simulink model "motor_testbench"  (R2021a)
settings: Solver=ode23t  StartTime=0.0  StopTime=0.1  RelTol=1e-3  AbsTol=1e-3  EnableMultiTasking=on
values from neighbouring files (symbols this model uses):
  f = n_rpm/60.0*p    (= 250)    [uz_6ph_pu_vsd_voltages_init.m]    (also in uz_mpc_6ph_init.m; uz_mpc_6ph_state_machine_init.m = 83.3333333333)
  IB = sqrt(2)*IR    [uz_6ph_pu_vsd_voltages_init.m]    (also in uz_mpc_6ph_init.m; uz_mpc_6ph_state_machine_init.m)
  id_ref = 0.0    (= 0)    [uz_6ph_pu_vsd_voltages_init.m]    (also in uz_mpc_6ph_init.m; uz_mpc_6ph_state_machine_init.m)
  iq_ref = -10.0    (= -10)    [uz_6ph_pu_vsd_voltages_init.m]    (also in uz_mpc_6ph_init.m; uz_mpc_6ph_state_machine_init.m = 5)
  ix_ref = 0.0    (= 0)    [uz_6ph_pu_vsd_voltages_init.m]    (also in uz_mpc_6ph_init.m; uz_mpc_6ph_state_machine_init.m)
  iy_ref = 0.0    (= 0)    [uz_6ph_pu_vsd_voltages_init.m]    (also in uz_mpc_6ph_init.m; uz_mpc_6ph_state_machine_init.m)
  lambda_d = 1.0    (= 1)    [uz_mpc_6ph_state_machine_init.m]
  lambda_q = 1.0    (= 1)    [uz_mpc_6ph_state_machine_init.m]
  lambda_u = 0.0    (= 0)    [uz_mpc_6ph_state_machine_init.m]
  lambda_x = 1.0    (= 1)    [uz_mpc_6ph_state_machine_init.m]
  lambda_y = 1.0    (= 1)    [uz_mpc_6ph_state_machine_init.m]
  Ld_over_LB = Ld/LB    [uz_6ph_pu_vsd_voltages_init.m]    (also in uz_mpc_6ph_init.m; uz_mpc_6ph_state_machine_init.m)
  Lq_over_LB = Lq/LB    [uz_6ph_pu_vsd_voltages_init.m]    (also in uz_mpc_6ph_init.m; uz_mpc_6ph_state_machine_init.m)
  omega_m = n_rpm*pi/30    (= 314.159265359)    [uz_6ph_pu_vsd_voltages_init.m]    (also in uz_mpc_6ph_init.m; uz_mpc_6ph_state_machine_init.m = 104.71975512)
  omegaB = nR*2*pi()/60*p    [uz_6ph_pu_vsd_voltages_init.m]    (also in uz_mpc_6ph_init.m; uz_mpc_6ph_state_machine_init.m)
  p = 5    [uz_6ph_pu_vsd_voltages_init.m]    (also in uz_mpc_6ph_init.m; uz_mpc_6ph_state_machine_init.m)
  psi_pm_over_psiB = psi_pm/psiB    [uz_6ph_pu_vsd_voltages_init.m]    (also in uz_mpc_6ph_init.m; uz_mpc_6ph_state_machine_init.m)
  Rs_over_ZB = Rs/ZB    [uz_6ph_pu_vsd_voltages_init.m]    (also in uz_mpc_6ph_init.m; uz_mpc_6ph_state_machine_init.m)
  t_ADC = 1/f_ADC    (= 1e-05)    [uz_6ph_pu_vsd_voltages_init.m]    (also in uz_mpc_6ph_init.m; uz_mpc_6ph_state_machine_init.m; uz_typeconv_init.m)
  t_clock = 1/f_clock    (= 1e-08)    [uz_6ph_pu_vsd_voltages_init.m]    (also in uz_mpc_6ph_init.m; uz_mpc_6ph_state_machine_init.m; uz_typeconv_init.m)
  Ts_times_ZB_over_Ld = Ts*ZB/Ld    [uz_6ph_pu_vsd_voltages_init.m]    (also in uz_mpc_6ph_init.m; uz_mpc_6ph_state_machine_init.m)
  Ts_times_ZB_over_Lq = Ts*ZB/Lq    [uz_6ph_pu_vsd_voltages_init.m]    (also in uz_mpc_6ph_init.m; uz_mpc_6ph_state_machine_init.m)
  Ts_times_ZB_over_Lx = Ts*ZB/Lx    [uz_6ph_pu_vsd_voltages_init.m]    (also in uz_mpc_6ph_init.m; uz_mpc_6ph_state_machine_init.m)
  Ts_times_ZB_over_Ly = Ts*ZB/Ly    [uz_6ph_pu_vsd_voltages_init.m]    (also in uz_mpc_6ph_init.m; uz_mpc_6ph_state_machine_init.m)
  v_dc = 565.0    (= 565)    [uz_6ph_pu_vsd_voltages_init.m]    (also in uz_mpc_6ph_init.m; uz_mpc_6ph_state_machine_init.m)
  VB = sqrt(2/3)*VR    [uz_6ph_pu_vsd_voltages_init.m]    (also in uz_mpc_6ph_init.m; uz_mpc_6ph_state_machine_init.m)
undefined symbols (not defined in the file or in its folder): Newton, Raphson
libraries: nesl_utility x33, fl_lib x26, ee_lib x12, simulink x10, hdlsllib x2, spsAlphaBetaZerotodq0Lib x1
(part 1 of 3)
settings Model: Creator=Michael Hoerner  LastModifiedBy=micha
settings SolverCC: AutoScaleAbsTol=off  AlgebraicLoopSolver=TrustRegion  DecoupledContinuousIntegration=on  MinimalZcImpactIntegration=on
settings DataIOCC: LimitDataPoints=on  MaxDataPoints=10000  ReturnWorkspaceOutputs=off
settings OptimizationCC: DefaultParameterBehavior=Inlined  PassReuseOutputArgsAs=Individual arguments  OptimizeBlockOrder=speed  DifferentSizesBufferReuse=on  EfficientTunableParamExpr=on
settings DebuggingCC: ParameterTunabilityLossMsg=error  AllowSymbolicDim=off  SFUnexpectedBacktrackingDiag=warning  SFNoUnconditionalDefaultTransitionDiag=warning  SFExecutionAtInitializationDiag=none  SFMachineParentedDataDiag=warning  ArithmeticOperatorsInVariantConditions=warning
settings HardwareCC: ProdBitPerPointer=32  ProdBitPerSizeT=32  ProdBitPerPtrDiffT=32  ProdLargestAtomicInteger=Long  ProdLargestAtomicFloat=Double  ProdWordSize=32  ProdHWDeviceType=ARM Compatible->ARM Cortex-R
settings SFSimCC: SimUseLocalCustomCode=off  MATLABDynamicMemAlloc=off  CustomCodeUndefinedFunction=UseInterfaceOnly
settings RTWCC: SystemTargetFile=ert.tlc  GenCodeOnly=on  TemplateMakefile=ert_default_tmf  GenerateReport=on  RTWUseLocalCustomCode=off  BuildConfiguration=Faster Runs  IncludeHyperlinkInReport=on  GenerateTraceInfo=on  GenerateTraceReport=on  GenerateTraceReportSl=on  GenerateTraceReportSf=on  GenerateTraceReportEml=on  GenerateCodeMetricsReport=on  CheckMdlBeforeBuild=Warning
settings CodeAppCC: ForceParamTrailComments=on  IgnoreCustomStorageClasses=off  OperatorAnnotations=on  SimulinkDataObjDesc=on  SFDataObjDesc=on  MATLABFcnDesc=on  InsertBlockDesc=on  StateflowObjectComments=on  MATLABSourceComments=on  EnableCustomComments=on  ReqsInCode=on
settings ERTTargetCC: CodeReplacementLibrary=GNU C99 extensions  GenerateSampleERTMain=on  SuppressErrorStatus=on  IncludeFileDelimiter=UseQuote  CodeInterfacePackaging=Reusable function  SupportNonFinite=off  MultiInstanceErrorCode=Warning  RootIOFormat=Part of model data structure  ERTCustomFileTemplate=example_file_process.tlc  GlobalDataDefinition=InSourceFile  GlobalDataReference=InSourceFile  ERTFilePackagingFormat=CompactWithDataFile
settings ConfigComp: CovMetricSettings=dw  CovSaveCumulativeToWorkspaceVar=on  CovSaveSingleToWorkspaceVar=on  CovExternalEMLEnable=off  CovSFcnEnable=off
settings SimscapeCC: SimscapeLogDataHistory=10000

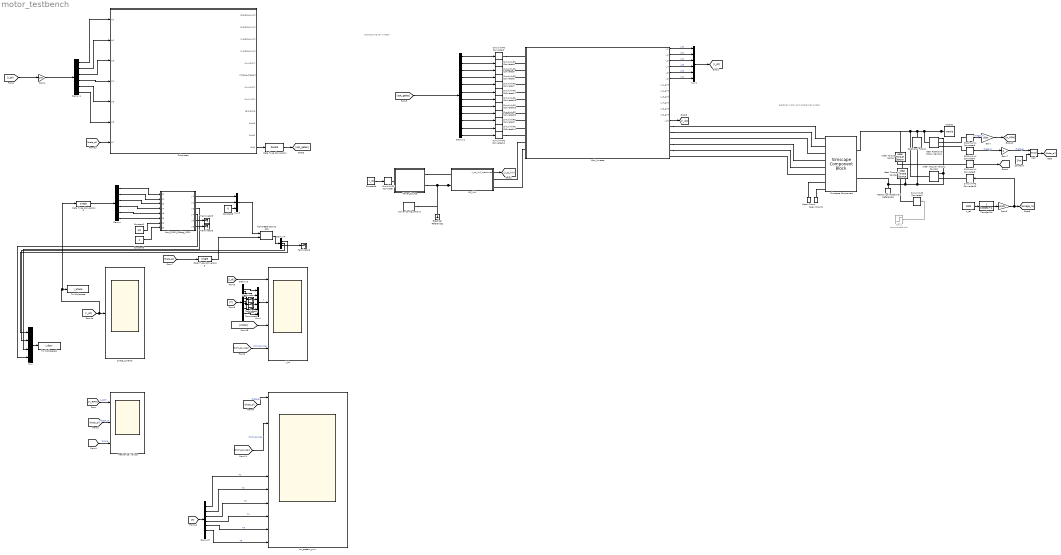
== system motor_testbench ==
  note: electrical motor and mechanical system
  note: 6-phase 2-level inverter
  6ph_Inverter : Subsystem
  6ph_PMSM_30deg_VSD1 : MATLAB Function  TreatAsAtomicUnit=on
  Alpha-Beta-Zero to dq0 : spsAlphaBetaZerotodq0Lib/Alpha-Beta-Zero to dq0  Alignment=Aligned with phase A axis
      settings: SourceProductBaseCode=PS
  Constant : Constant  Value=2*pi
  Constant1 : Constant  Value=1/3
  Constant6 : Constant  Value=v_dc
  Constant8 : Constant  Value=0  OutDataTypeStr=single
  Constant9 : Constant
  DC_link : Subsystem
  Data Type Conversion : DataTypeConversion  OutDataTypeStr=double  LockScale=on
  Data Type Conversion5 : DataTypeConversion  OutDataTypeStr=single
  Data Type Conversion6 : DataTypeConversion  OutDataTypeStr=single
  Demux : Demux  Outputs=6
  Demux1 : Demux  Outputs=6
  Demux2 : Demux  Outputs=12
  Demux3 : Demux  Outputs=12
  Demux4 : Demux  Outputs=3
  Demux5 : Demux  Outputs=12
  Electrical Reference1 : fl_lib/Electrical/Electrical Elements/Electrical Reference
  Gain : Gain  Gain=30/pi
  Gain1 : Gain  Gain=1/IB
  Gain7 : Gain  Gain=p
  Gain8 : Gain  Gain=pi/30
  Ideal Angular Velocity Source1 : fl_lib/Mechanical/Mechanical Sources/Ideal Angular Velocity Source
  Ideal Rotational Motion Sensor1 : fl_lib/Mechanical/Mechanical Sensors/Ideal Rotational Motion Sensor  wrap_angle=simscape.enum.onoff.off  offset=0 deg
  Ideal Torque Sensor : fl_lib/Mechanical/Mechanical Sensors/Ideal Torque Sensor
  Ideal Torque Source : fl_lib/Mechanical/Mechanical Sources/Ideal Torque Source
  Inertia1 : fl_lib/Mechanical/Rotational Elements/Inertia  inertia=J kg*m^2  num_ports=foundation.enum.numPorts2.one  w_specify=off  w_priority=High  w=0 rad/s  w_nominal_specify=off  w_nominal_unit=rad/s  w_nominal_value=1  t_specify=off  t_priority=None  t=0 N*m  t_nominal_specify=off  t_nominal_unit=N*m  t_nominal_value=1
  Mechanical Rotational Reference1 : fl_lib/Mechanical/Rotational Elements/Mechanical Rotational Reference
  Mod : Math  Operator=mod  SaturateOnIntegerOverflow=on
  Mux : Mux
  Mux1 : Mux  Inputs=6
  Mux4 : Mux  Inputs=6
  Mux5 : Mux  Inputs=3
  Open Circuit : fl_lib/Electrical/Electrical Elements/Open Circuit  v_specify=off  v_priority=None  v=0 V  v_nominal_specify=off  v_nominal_unit=V  v_nominal_value=1
      settings: SourceProductBaseCode=SS
  Open Circuit1 : fl_lib/Electrical/Electrical Elements/Open Circuit  v_specify=off  v_priority=None  v=0 V  v_nominal_specify=off  v_nominal_unit=V  v_nominal_value=1
      settings: SourceProductBaseCode=SS
  PS-Simulink Converter6 : nesl_utility/PS-Simulink Converter  PhysicalDomain=network_engine_domain  SubClassName=ps_output  LeftPortType=input  RightPortType=output  PseudoPeriodic=off  Frequencies=[]  Unit=1  AffineConversion=off
      settings: SourceProductBaseCode=PW,SS
  PS-Simulink Converter7 : nesl_utility/PS-Simulink Converter  PhysicalDomain=network_engine_domain  SubClassName=ps_output  LeftPortType=input  RightPortType=output  PseudoPeriodic=off  Frequencies=[]  Unit=1  AffineConversion=off
      settings: SourceProductBaseCode=PW,SS
  PS-Simulink Converter8 : nesl_utility/PS-Simulink Converter  PhysicalDomain=network_engine_domain  SubClassName=ps_output  LeftPortType=input  RightPortType=output  PseudoPeriodic=off  Frequencies=[]  Unit=1  AffineConversion=off
      settings: SourceProductBaseCode=PW,SS
  Power_Source : Subsystem
  Rotational Friction : fl_lib/Mechanical/Rotational Elements/Rotational Friction  brkwy_trq=0.0622476 N*m  brkwy_vel=0.1 rad/s  Col_trq=0.03460117 N*m  visc_coef=0.00026373 N*m/(rad/s)  w_specify=off  w_priority=None  w=0 rad/s  w_nominal_specify=off  w_nominal_unit=rad/s  w_nominal_value=1  t_specify=off  t_priority=None  t=0 N*m  t_nominal_specify=off  t_nominal_unit=N*m  t_nominal_value=1
  Simscape Component : SimscapeComponentBlock  SourceFile=SixPhase_PMSM  ComponentPath=SixPhase_PMSM  ComponentVariants=SixPhase_PMSM  ComponentVariantNames=SixPhase_PMSM  ClassName=SixPhase_PMSM  SchemaVersion=1  Rs=Rs Ohm  Ld=Ld H  Lq=Lq H  Lx=Lx H  Ly=Ly H  psiPM=psi_pm Wb  np=p  theta_m_specify=off  theta_m_priority=None  theta_m=0 rad  theta_m_nominal_specify=off  theta_m_nominal_unit=rad  theta_m_nominal_value=1
      settings: CopyFcn=simscape.engine.sli.internal.componentblockcallback(gcbh,'COPY')  PreCopyFcn=simscape.engine.sli.internal.componentblockcallback(gcbh,'PRECOPY')  PreDeleteFcn=simscape.engine.sli.internal.componentblockcallback(gcbh,'PREDELETE')  InternalSimscapePortConfiguration="{\"Bottom\":[],\"Left\":[{\"id\":\"a1\",\"label\":\"a1\",\"type\":\"foundation.electrical.electrical\"},{\"id\":\"b1\",\"label\":\"b1\",\"type\":\"foundation.electrical.electrical\"},{\"id\":\"c1\",\"label\":\"c1\",\"type\":\"foundation.electrical.electrical\"},{\"id\":\"a2\",\"label\":\"a2\",\"type\":\"foundation.electrical.electrical\"},{\"id\":\"b2\",\"label\":\"b2\",\"type\":\"foundation.electrical.electrical\"},{\"id\":\"c2\",\"label\":\"c2\",\"type\":\"foundation.electrical.electrical\"},{\"id\":\"n1\",\"label\":\"n1\",\"type\":\"foundation.electrical.electrical\"},{\"id\":\"n2\",\"label\":\"n2\",\"type\":\"foundation.electrical.electrical\"}],\"Right\":[{\"id\":\"R\",\"label\":\"R\",\"type\":\"foundation.mechanical.rotational.rotational\"},{\"id\":\"C\",\"label\":\"C\",\"type\":\"foundation.mechanical.rotational.rotational\"}],\"Top\":[]}"
      mask Type: SixPhase_PMSM
  Simulink-PS Converter{,2..7,11..12,17..20} (13 alike) : nesl_utility/Simulink-PS Converter  PhysicalDomain=network_engine_domain  SubClassName=ps_input  LeftPortType=input  RightPortType=output  PseudoPeriodic=off  Frequencies=[]  NoiseDistribution=none  NoiseParameters=[]  Unit=1  AffineConversion=off  FilteringAndDerivatives=provide  SimscapeFilterOrder=1  InputFilterTimeConstant=0.001  UdotUserProvided=0
      Simulink-PS Converter settings: SourceProductBaseCode=PW,SS
  Simulink-PS Converter1 : nesl_utility/Simulink-PS Converter  PhysicalDomain=network_engine_domain  SubClassName=ps_input  LeftPortType=input  RightPortType=output  PseudoPeriodic=off  Frequencies=[]  NoiseDistribution=none  NoiseParameters=[]  Unit=1  AffineConversion=off  FilteringAndDerivatives=filter  SimscapeFilterOrder=1  InputFilterTimeConstant=0.001  UdotUserProvided=0
      settings: SourceProductBaseCode=PW,SS
  Simulink-PS Converter10 : nesl_utility/Simulink-PS Converter  PhysicalDomain=network_engine_domain  SubClassName=ps_input  LeftPortType=input  RightPortType=output  PseudoPeriodic=off  Frequencies=[]  NoiseDistribution=none  NoiseParameters=[]  Unit=1  AffineConversion=off  FilteringAndDerivatives=filter  SimscapeFilterOrder=1  InputFilterTimeConstant=0.001  UdotUserProvided=0
      settings: SourceProductBaseCode=PW,SS
  Solver Configuration1 : nesl_utility/Solver Configuration  PhysicalDomain=network_engine_domain  SubClassName=solver  LeftPortType=input  RightPortType=generic  Tones=[]  Harmonics=[]  SimulateNoise=off  Profile=off  UseLocalSampling=off  EnableSwitchedLinearOptims=on  FrequencyDomain=off  UseCCode=off  RelTol=0.001  AbsTol=1e-06  MinStep=1e-09  ToWorkspace=off  RevertToSquareIcSolve=off  NumHomotopyIterations=100  PhasorMode=off  PhasorModeNumHarmonics=1  DoDC=off  ResidualTolerance=1e-09  UseLocalSolver=off  LocalSolverChoice=NE_BACKWARD_EULER_ADVANCER  LocalSolverSampleTime=1e-6  DoFixedCost=off  MaxNonlinIter=3  MaxModeIter=2  ComputeImpulses=off  ImpulseIterations=2  LinearAlgebra=Sparse  EquationFormulation=NE_TIME_EF  DelaysMemoryBudget=1024  AutomaticFiltering=on  FilteringTimeConstant=0.001  PartitionStorageMethod=AS_NEEDED  PartitionMemoryBudget=1024  PartitionMethod=FAST
      settings: SourceProductBaseCode=PW,SS
  Step1 : Step  Commented=on  Time=0.08  After=-0.5  SampleTime=0
  Subsystem : Subsystem
  Terminator{,1..3,5..6} (6 alike) : Terminator
  To Workspace : ToWorkspace  VariableName=i_phase  SaveFormat=Timeseries  SampleTime=1e-6
  To Workspace1 : ToWorkspace  VariableName=i_dqxy  SaveFormat=Timeseries  SampleTime=50e-6
  Transfer Fcn : TransferFcn  Denominator=[0.0005 1]
  i_dc : Scope  NumInputPorts=4
  mechanical values : Scope  NumInputPorts=3
  n_ref : Constant  Value=1000
  phase_currents : Scope
  sw_pattern_svm : Scope  NumInputPorts=12
  wires:
  DC_link/1(u_dc_link_measured) -> [u_dc_link]
  Constant6/1 -> Simulink-PS Converter/1
  PS-Simulink Converter7/1 -> Gain7/1  "theta_m"
  Gain7/1 -> Mod/1  "theta_el"
  Gain8/1 -> Simulink-PS Converter10/1, [omega_m]
  PS-Simulink Converter6/1 -> Gain/1  "omega_m"
  PS-Simulink Converter8/1 -> [torque]
  [T] -> Demux3/1
  Demux3/1 -> Mux4/1
  Demux3/3 -> Mux4/2
  Demux3/5 -> Mux4/3
  Demux3/2 -> Terminator/1
  Demux3/4 -> Terminator1/1
  [PWM_counter] -> i_dc/4  "PWM_counter"
  [i_dc] -> i_dc/1
  Demux3/6 -> Terminator3/1
  [i_ph] -> Data Type Conversion6/1, To Workspace/1, phase_currents/1
  Mux4/1 -> i_dc/2  "T"
  n_ref/1 -> Transfer Fcn/1
  Transfer Fcn/1 -> Gain8/1
  [CMPA] -> i_dc/3
  Gain/1 -> [n_RPM]
  Step1/1 -> Simulink-PS Converter1/1
  [torque] -> mechanical values/3  "torque"
  [n_RPM] -> mechanical values/1  "n_RPM"
  [theta_el] -> mechanical values/2  "theta_el"
  6ph_Inverter/1(i_1) -> Mux1/1  "i_a1"
  6ph_Inverter/6(i_6) -> Mux1/6  "i_c2"
  6ph_Inverter/4(i_4) -> Mux1/4  "i_a2"
  Demux2/6 -> Simulink-PS Converter17/1
  Demux2/5 -> Simulink-PS Converter7/1
  6ph_Inverter/13(i_dc) -> [i_dc]
  Demux2/7 -> Simulink-PS Converter18/1
  6ph_Inverter/3(i_3) -> Mux1/3  "i_c1"
  6ph_Inverter/5(i_5) -> Mux1/5  "i_b2"
  Demux2/3 -> Simulink-PS Converter5/1
  6ph_Inverter/2(i_2) -> Mux1/2  "i_b1"
  Demux2/2 -> Simulink-PS Converter4/1
  Demux2/11 -> Simulink-PS Converter11/1
  Demux2/12 -> Simulink-PS Converter12/1
  Demux2/8 -> Simulink-PS Converter19/1
  Demux2/9 -> Simulink-PS Converter20/1
  Demux2/4 -> Simulink-PS Converter6/1
  Demux2/10 -> Simulink-PS Converter3/1
  Demux2/1 -> Simulink-PS Converter2/1
  Mux1/1 -> [i_ph]
  Constant/1 -> Mod/2
  Mod/1 -> [theta_el]
  Mux/1 -> To Workspace1/1
  6ph_PMSM_30deg_VSD1/3(y3) -> Mux/3
  Demux/2 -> 6ph_PMSM_30deg_VSD1/2(u2)
  Constant8/1 -> Mux5/3
  Constant9/1 -> 6ph_PMSM_30deg_VSD1/8(c6)
  Demux/5 -> 6ph_PMSM_30deg_VSD1/5(u5)
  Demux/4 -> 6ph_PMSM_30deg_VSD1/4(u4)
  Demux/6 -> 6ph_PMSM_30deg_VSD1/6(u6)
  6ph_PMSM_30deg_VSD1/2(y2) -> Mux5/2
  6ph_PMSM_30deg_VSD1/6(y6) -> Terminator6/1
  Demux/3 -> 6ph_PMSM_30deg_VSD1/3(u3)
  Constant1/1 -> 6ph_PMSM_30deg_VSD1/7(k6)
  Demux/1 -> 6ph_PMSM_30deg_VSD1/1(u1)
  6ph_PMSM_30deg_VSD1/4(y4) -> Mux/4
  Mux5/1 -> Alpha-Beta-Zero to dq0/1
  6ph_PMSM_30deg_VSD1/5(y5) -> Terminator5/1
  6ph_PMSM_30deg_VSD1/1(y1) -> Mux5/1
  [theta_el] -> Data Type Conversion5/1
  Alpha-Beta-Zero to dq0/1 -> Demux4/1
  Demux4/1 -> Mux/1
  Demux4/2 -> Mux/2
  Demux4/3 -> Terminator2/1
  Data Type Conversion5/1 -> Alpha-Beta-Zero to dq0/2
  Data Type Conversion6/1 -> Demux/1
  Demux3/11 -> Mux4/6
  Demux3/9 -> Mux4/5
  Demux3/7 -> Mux4/4
  [theta_el] -> sw_pattern_svm/1  "theta_el"
  [PWM_counter] -> sw_pattern_svm/3  "PWM_counter"
  Demux5/7 -> sw_pattern_svm/10  "T4"
  Demux5/3 -> sw_pattern_svm/8  "T2"
  Demux5/9 -> sw_pattern_svm/11  "T5"
  [T] -> Demux5/1
  Demux5/1 -> sw_pattern_svm/7  "T1"
  Demux5/5 -> sw_pattern_svm/9  "T3"
  Demux5/11 -> sw_pattern_svm/12  "T6"
  [opt_gates] -> Demux2/1
  Subsystem/12(Out1) -> Data Type Conversion/1
  Data Type Conversion/1 -> [opt_gates]
  Demux1/1 -> Subsystem/1(In1)
  [i_ph] -> Gain1/1
  Gain1/1 -> Demux1/1
  Demux1/2 -> Subsystem/2(In2)
  Demux1/3 -> Subsystem/3(In3)
  Demux1/4 -> Subsystem/4(In4)
  Demux1/5 -> Subsystem/5(In5)
  Demux1/6 -> Subsystem/6(In6)
  [theta_el] -> Subsystem/7(In7)
  connections:
  DC_link/LConn2 -- Power_Source/RConn2 -- Solver Configuration1/RConn1 -- Electrical Reference1/LConn1
  Inertia1/LConn1 -- Ideal Torque Sensor/LConn1 -- Simscape Component/RConn1 -- Ideal Angular Velocity Source1/LConn1 -- Rotational Friction/LConn1 -- Ideal Rotational Motion Sensor1/LConn1
  Ideal Rotational Motion Sensor1/RConn1 -- Ideal Angular Velocity Source1/RConn2 -- Rotational Friction/RConn1 -- Simscape Component/RConn2 -- Mechanical Rotational Reference1/LConn1 -- Ideal Torque Source/RConn2
  Power_Source/RConn1 -- DC_link/LConn1
  PS-Simulink Converter6/LConn1 -- Ideal Rotational Motion Sensor1/RConn2
  Simulink-PS Converter/RConn1 -- Power_Source/LConn1
  6ph_Inverter/LConn13 -- DC_link/RConn1
  6ph_Inverter/LConn14 -- DC_link/RConn2
  PS-Simulink Converter7/LConn1 -- Ideal Rotational Motion Sensor1/RConn3
  Simulink-PS Converter10/RConn1 -- Ideal Angular Velocity Source1/RConn1
  PS-Simulink Converter8/LConn1 -- Ideal Torque Sensor/RConn2
  Simulink-PS Converter1/RConn1 -- Ideal Torque Source/RConn1
  Ideal Torque Source/LConn1 -- Ideal Torque Sensor/RConn1
  Simscape Component/LConn8 -- Open Circuit1/LConn1
  6ph_Inverter/RConn2 -- Simscape Component/LConn2
  Simscape Component/LConn7 -- Open Circuit/LConn1
  6ph_Inverter/RConn1 -- Simscape Component/LConn1
  6ph_Inverter/RConn4 -- Simscape Component/LConn4
  6ph_Inverter/RConn5 -- Simscape Component/LConn5
  Simulink-PS Converter7/RConn1 -- 6ph_Inverter/LConn5
  Simulink-PS Converter12/RConn1 -- 6ph_Inverter/LConn12
  Simulink-PS Converter20/RConn1 -- 6ph_Inverter/LConn9
  Simulink-PS Converter17/RConn1 -- 6ph_Inverter/LConn6
  Simulink-PS Converter11/RConn1 -- 6ph_Inverter/LConn11
  Simulink-PS Converter19/RConn1 -- 6ph_Inverter/LConn8
  Simulink-PS Converter6/RConn1 -- 6ph_Inverter/LConn4
  Simulink-PS Converter3/RConn1 -- 6ph_Inverter/LConn10
  Simulink-PS Converter4/RConn1 -- 6ph_Inverter/LConn2
  Simscape Component/LConn3 -- 6ph_Inverter/RConn3
  Simscape Component/LConn6 -- 6ph_Inverter/RConn6
  Simulink-PS Converter5/RConn1 -- 6ph_Inverter/LConn3
  Simulink-PS Converter2/RConn1 -- 6ph_Inverter/LConn1
  Simulink-PS Converter18/RConn1 -- 6ph_Inverter/LConn7

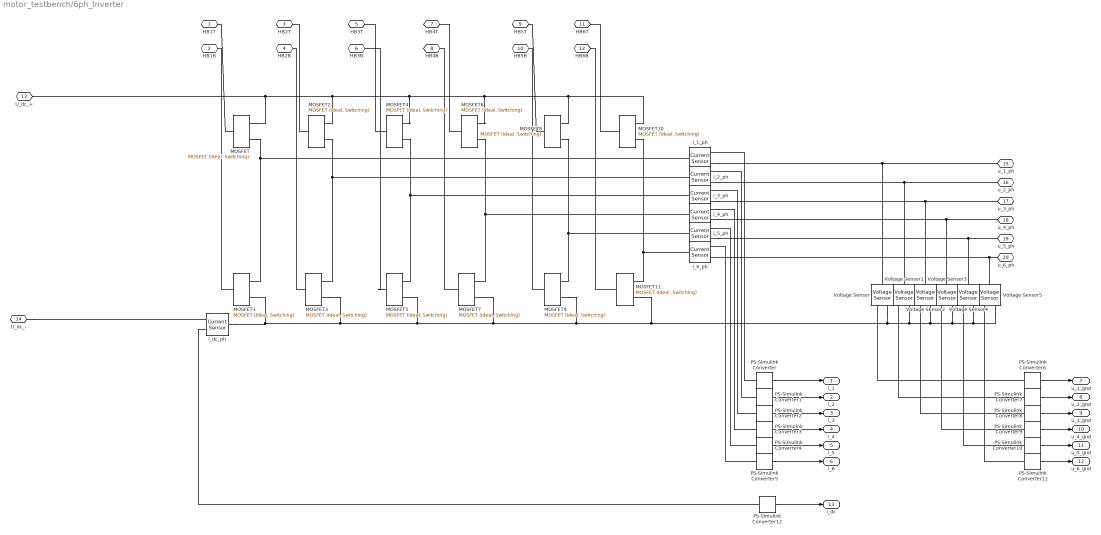
== system motor_testbench/6ph_Inverter ==
  MOSFET{,1..11} (12 alike) : ee_lib/Semiconductors & Converters/MOSFET (Ideal, Switching)  Rds=RDSon Ohm  Goff=1e-6 1/Ohm  Vth=0.7 V  diode_param=1  diode_Vf=0.8 V  diode_Ron=0.001 Ohm  diode_Goff=1e-5 1/Ohm  diode_C=5e-8 F  diode_iRM=-235 A  diode_iF=300 A  diode_idot=-50 A/us  diode_trr_param=1  diode_trr_factor=3  diode_trr=15 us  diode_Qrr=1.5e+3 s*uA  thermal_loss_option=ee.enum.converters.thermalLossOption.constantvalues  Von_data=[0, 1.1, 1.3, 1.45, 1.75, 2.25, 2.7; 0, 1, 1.15, 1.35, 1.7, 2.35, 3] V  Eon_data=[0, .29, 1.43, 2.86, 5.71, 13.14, 22.86; 0, .57, 2.63, 5.14, 10.29, 20.57, 30.29] * 1e-3 J  Eoff_data=[0, .21, 1.07, 2.14, 4.29, 9.86, 17.14; 0, .43, 1.97, 3.86, 7.71, 15.43, 22.71] * 1e-3 J  Tj=[298.15, 398.15] K  Iout_data=[0, 10, 50, 100, 200, 400, 600] A  Eon_scalar=22.86e-3 J  Eoff_scalar=17.14e-3 J  Voff=300 V  Iout_scalar=600 A  diodeModelType=ee.enum.converters.diodeModelType.pwl  diode_IfMat=[.07, .12, .19, 1.75, 4.24, 7.32, 11.2; .16, .3, .72, 2.14, 4.02, 6.35, 9.12] A  diode_TjVec=[25, 125] degC  diode_VfVec=[.5, .7, .9, 1.3, 1.7, 2.1, 2.5] V  thermal_network_parameterization=ee.enum.thermalNetworkTopology.external  Rth=[.03, .2] K/W  Rth_Foster=[.03, .2] K/W  thermal_mass_parameterization=ee.enum.thermalNetwork.timeconstant  thermal_mass=[3, 25] J/K  thermal_mass_Foster=[33, 50] J/K  thermal_time_constant=[.1, 5] s  thermal_time_constant_Foster=[1, 10] s  thermal_mass_initial_temperatures=[25, 25] degC  junction_thermal_mass=0.1 J/K  vT_specify=off  vT_priority=None  vT=0 V  vT_nominal_specify=off  vT_nominal_unit=V  vT_nominal_value=1  Qj_specify=off  Qj_priority=None  Qj=0 W  Qj_nominal_specify=off  Qj_nominal_unit=W  Qj_nominal_value=1  junction_temperature_specify=off  junction_temperature_priority=None  junction_temperature=25 degC  junction_temperature_nominal_specify=off  junction_temperature_nominal_unit=degC  junction_temperature_nominal_value=1
  PS-Simulink Converter{,1..5,12} (7 alike) : nesl_utility/PS-Simulink Converter  PhysicalDomain=network_engine_domain  SubClassName=ps_output  LeftPortType=input  RightPortType=output  PseudoPeriodic=off  Frequencies=[]  Unit=A  AffineConversion=off
  PS-Simulink Converter{6..11} (6 alike) : nesl_utility/PS-Simulink Converter  PhysicalDomain=network_engine_domain  SubClassName=ps_output  LeftPortType=input  RightPortType=output  PseudoPeriodic=off  Frequencies=[]  Unit=V  AffineConversion=off
  Voltage Sensor{,1..5} (6 alike) : fl_lib/Electrical/Electrical Sensors/Voltage Sensor
  i_1_ph : fl_lib/Electrical/Electrical Sensors/Current Sensor
  i_2_ph : fl_lib/Electrical/Electrical Sensors/Current Sensor
  i_3_ph : fl_lib/Electrical/Electrical Sensors/Current Sensor
  i_4_ph : fl_lib/Electrical/Electrical Sensors/Current Sensor
  i_5_ph : fl_lib/Electrical/Electrical Sensors/Current Sensor
  i_6_ph : fl_lib/Electrical/Electrical Sensors/Current Sensor
  i_dc_ph : fl_lib/Electrical/Electrical Sensors/Current Sensor
  HB1T : PMIOPort  Side=Left
  HB1B : PMIOPort  Port=2  Side=Left
  HB2T : PMIOPort  Port=3  Side=Left
  HB2B : PMIOPort  Port=4  Side=Left
  HB3T : PMIOPort  Port=5  Side=Left
  HB3B : PMIOPort  Port=6  Side=Left
  HB4T : PMIOPort  Port=7  Side=Left
  HB4B : PMIOPort  Port=8  Side=Left
  HB5T : PMIOPort  Port=9  Side=Left
  HB5B : PMIOPort  Port=10  Side=Left
  HB6T : PMIOPort  Port=11  Side=Left
  HB6B : PMIOPort  Port=12  Side=Left
  U_dc_+ : PMIOPort  Port=13  Side=Left
  U_dc_- : PMIOPort  Port=14  Side=Left
  u_1_ph : PMIOPort  Port=15  Side=Right
  u_2_ph : PMIOPort  Port=16  Side=Right
  u_3_ph : PMIOPort  Port=17  Side=Right
  u_4_ph : PMIOPort  Port=18  Side=Right
  u_5_ph : PMIOPort  Port=19  Side=Right
  u_6_ph : PMIOPort  Port=20  Side=Right
  i_1 : Outport  VectorParamsAs1DForOutWhenUnconnected=off
  i_2 : Outport  Port=2  VectorParamsAs1DForOutWhenUnconnected=off
  i_3 : Outport  Port=3  VectorParamsAs1DForOutWhenUnconnected=off
  i_4 : Outport  Port=4  VectorParamsAs1DForOutWhenUnconnected=off
  i_5 : Outport  Port=5  VectorParamsAs1DForOutWhenUnconnected=off
  i_6 : Outport  Port=6  VectorParamsAs1DForOutWhenUnconnected=off
  u_1_gnd : Outport  Port=7  VectorParamsAs1DForOutWhenUnconnected=off
  u_2_gnd : Outport  Port=8  VectorParamsAs1DForOutWhenUnconnected=off
  u_3_gnd : Outport  Port=9  VectorParamsAs1DForOutWhenUnconnected=off
  u_4_gnd : Outport  Port=10  VectorParamsAs1DForOutWhenUnconnected=off
  u_5_gnd : Outport  Port=11  VectorParamsAs1DForOutWhenUnconnected=off
  u_6_gnd : Outport  Port=12  VectorParamsAs1DForOutWhenUnconnected=off
  i_dc : Outport  Port=13  VectorParamsAs1DForOutWhenUnconnected=off
  wires:
  PS-Simulink Converter/1 -> i_1/1
  PS-Simulink Converter1/1 -> i_2/1
  PS-Simulink Converter2/1 -> i_3/1
  PS-Simulink Converter3/1 -> i_4/1
  PS-Simulink Converter4/1 -> i_5/1
  PS-Simulink Converter5/1 -> i_6/1
  PS-Simulink Converter9/1 -> u_4_gnd/1
  PS-Simulink Converter8/1 -> u_3_gnd/1
  PS-Simulink Converter7/1 -> u_2_gnd/1
  PS-Simulink Converter6/1 -> u_1_gnd/1
  PS-Simulink Converter10/1 -> u_5_gnd/1
  PS-Simulink Converter11/1 -> u_6_gnd/1
  PS-Simulink Converter12/1 -> i_dc/1
  connections:
  MOSFET6/RConn2 -- i_4_ph/LConn1 -- MOSFET7/RConn1
  MOSFET2/RConn2 -- i_2_ph/LConn1 -- MOSFET3/RConn1
  MOSFET4/RConn2 -- i_3_ph/LConn1 -- MOSFET5/RConn1
  MOSFET5/RConn2 -- Voltage Sensor5/RConn2 -- Voltage Sensor4/RConn2 -- Voltage Sensor3/RConn2 -- Voltage Sensor2/RConn2 -- Voltage Sensor1/RConn2 -- Voltage Sensor/RConn2 -- MOSFET11/RConn2 -- MOSFET9/RConn2 -- MOSFET7/RConn2 -- i_dc_ph/LConn1 -- MOSFET1/RConn2 -- MOSFET3/RConn2
  MOSFET/RConn2 -- i_1_ph/LConn1 -- MOSFET1/RConn1
  MOSFET11/LConn1 -- HB6B/RConn1
  MOSFET8/RConn2 -- i_5_ph/LConn1 -- MOSFET9/RConn1
  MOSFET2/LConn1 -- HB2T/RConn1
  MOSFET10/RConn2 -- i_6_ph/LConn1 -- MOSFET11/RConn1
  MOSFET/LConn1 -- HB1T/RConn1
  MOSFET9/LConn1 -- HB5B/RConn1
  MOSFET5/LConn1 -- HB3B/RConn1
  MOSFET1/LConn1 -- HB1B/RConn1
  MOSFET7/LConn1 -- HB4B/RConn1
  MOSFET8/LConn1 -- HB5T/RConn1
  MOSFET4/LConn1 -- HB3T/RConn1
  MOSFET10/LConn1 -- HB6T/RConn1
  MOSFET6/LConn1 -- HB4T/RConn1
  MOSFET3/LConn1 -- HB2B/RConn1
  i_1_ph/RConn2 -- Voltage Sensor/LConn1 -- u_1_ph/RConn1
  i_2_ph/RConn2 -- u_2_ph/RConn1 -- Voltage Sensor1/LConn1
  i_3_ph/RConn2 -- u_3_ph/RConn1 -- Voltage Sensor2/LConn1
  i_4_ph/RConn2 -- Voltage Sensor3/LConn1 -- u_4_ph/RConn1
  i_5_ph/RConn2 -- Voltage Sensor4/LConn1 -- u_5_ph/RConn1
  u_6_ph/RConn1 -- i_6_ph/RConn2 -- Voltage Sensor5/LConn1
  PS-Simulink Converter/LConn1 -- i_1_ph/RConn1
  PS-Simulink Converter1/LConn1 -- i_2_ph/RConn1
  PS-Simulink Converter2/LConn1 -- i_3_ph/RConn1
  i_4_ph/RConn1 -- PS-Simulink Converter3/LConn1
  PS-Simulink Converter4/LConn1 -- i_5_ph/RConn1
  PS-Simulink Converter5/LConn1 -- i_6_ph/RConn1
  PS-Simulink Converter6/LConn1 -- Voltage Sensor/RConn1
  PS-Simulink Converter7/LConn1 -- Voltage Sensor1/RConn1
  PS-Simulink Converter8/LConn1 -- Voltage Sensor2/RConn1
  PS-Simulink Converter9/LConn1 -- Voltage Sensor3/RConn1
  PS-Simulink Converter10/LConn1 -- Voltage Sensor4/RConn1
  PS-Simulink Converter11/LConn1 -- Voltage Sensor5/RConn1
  U_dc_-/RConn1 -- i_dc_ph/RConn2
  PS-Simulink Converter12/LConn1 -- i_dc_ph/RConn1
  MOSFET6/RConn1 -- MOSFET/RConn1 -- U_dc_+/RConn1 -- MOSFET2/RConn1 -- MOSFET4/RConn1 -- MOSFET10/RConn1 -- MOSFET8/RConn1

== system motor_testbench/DC_link ==
  Capacitor : fl_lib/Electrical/Electrical Elements/Capacitor  c=C_dc_link uF  r=1e-6 Ohm  g=0 1/Ohm  i_specify=off  i_priority=None  i=0 A  i_nominal_specify=off  i_nominal_unit=A  i_nominal_value=1  v_specify=off  v_priority=None  v=0 V  v_nominal_specify=off  v_nominal_unit=V  v_nominal_value=1  vc_specify=off  vc_priority=High  vc=0 V  vc_nominal_specify=off  vc_nominal_unit=V  vc_nominal_value=1
  PS-Simulink Converter : nesl_utility/PS-Simulink Converter  PhysicalDomain=network_engine_domain  SubClassName=ps_output  LeftPortType=input  RightPortType=output  PseudoPeriodic=off  Frequencies=[]  Unit=1  AffineConversion=off
      settings: SourceProductBaseCode=PW,SS
  Voltage Sensor : fl_lib/Electrical/Electrical Sensors/Voltage Sensor
  U_dc_link+_in : PMIOPort  Side=Left
  U_dc_link-_in : PMIOPort  Port=2  Side=Left
  U_dc_link+_out : PMIOPort  Port=3  Side=Right
  U_dc_link-_out : PMIOPort  Port=4  Side=Right
  u_dc_link_measured : Outport  VectorParamsAs1DForOutWhenUnconnected=off
  wires:
  PS-Simulink Converter/1 -> u_dc_link_measured/1
  connections:
  U_dc_link+_in/RConn1 -- Voltage Sensor/LConn1 -- U_dc_link+_out/RConn1 -- Capacitor/LConn1
  U_dc_link-_in/RConn1 -- Voltage Sensor/RConn2 -- U_dc_link-_out/RConn1 -- Capacitor/RConn1
  Voltage Sensor/RConn1 -- PS-Simulink Converter/LConn1

== system motor_testbench/Power_Source ==
  Controlled Voltage Source : fl_lib/Electrical/Electrical Sources/Controlled Voltage Source
  + : PMIOPort  Side=Right
  - : PMIOPort  Port=2  Side=Right
  ref_voltage : PMIOPort  Port=3  Side=Left
  connections:
  Controlled Voltage Source/LConn1 -- +/RConn1
  Controlled Voltage Source/RConn2 -- -/RConn1
  Controlled Voltage Source/RConn1 -- ref_voltage/RConn1

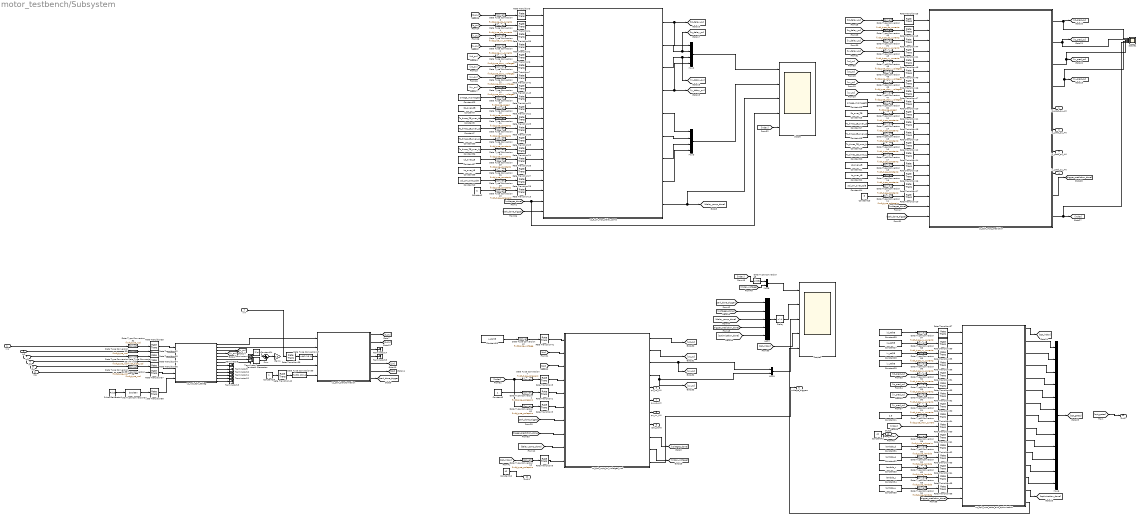
== system motor_testbench/Subsystem ==
  In1 : Inport
  In2 : Inport  Port=2
  In3 : Inport  Port=3
  In4 : Inport  Port=4
  In5 : Inport  Port=5
  In6 : Inport  Port=6
  In7 : Inport  Port=7
  Constant10 : Constant  Value=psi_pm_over_psiB
  Constant11 : Constant  Value=2.5
  Constant12 : Constant  Value=42
  Constant13 : Constant  Value=5
  Constant14 : Constant  Value=psi_pm_over_psiB
  Constant15 : Constant  Value=Rs_over_ZB
  Constant16 : Constant  Value=omega_m/omegaB
  Constant17 : Constant  Value=Ts_times_ZB_over_Ld
  Constant18 : Constant  Value=Ts_times_ZB_over_Lq
  Constant19 : Constant  Value=Ts_times_ZB_over_Lx
  Constant2 : Constant  Value=5
  Constant20 : Constant  Value=Ts_times_ZB_over_Ly
  Constant21 : Constant  Value=Ld_over_LB
  Constant22 : Constant  Value=Lq_over_LB
  Constant23 : Constant  Value=omega_m/omegaB
  Constant24 : Constant  Value=2*pi
  Constant25 : Constant
  Constant26 : Constant  Value=v_dc/VB
  Constant27 : Constant  Value=iq_ref/IB
  Constant28 : Constant  Value=ix_ref/IB
  Constant29 : Constant  Value=iy_ref/IB
  Constant3 : Constant
  Constant30 : Constant  Value=Ts_times_ZB_over_Lx
  Constant31 : Constant  Value=lambda_d
  Constant32 : Constant  Value=lambda_q
  Constant33 : Constant  Value=lambda_x
  Constant34 : Constant  Value=lambda_y
  Constant35 : Constant  Value=lambda_u
  Constant36 : Constant  Value=Ts_times_ZB_over_Ly
  Constant37 : Constant  Value=Ld_over_LB
  Constant38 : Constant  Value=Lq_over_LB
  Constant39 : Constant  Value=id_ref/IB
  Constant4 : Constant  Value=Rs_over_ZB
  Constant42 : Constant  Value=42
  Constant5 : Constant  Value=Ts_times_ZB_over_Ld
  Constant7 : Constant  Value=Ts_times_ZB_over_Lq
  Data Type Conversion{,2,31,43,50..51,55..58} (10 alike) : DataTypeConversion  OutDataTypeStr=fixdt_type_xy_currents
  Data Type Conversion{1,7,10..11,13,59,66} (7 alike) : DataTypeConversion  OutDataTypeStr=fixdt_type_polepairs
  Data Type Conversion{12,14..28} (16 alike) : DataTypeConversion  OutDataTypeStr=fixdt_type_constants
  Data Type Conversion29 : DataTypeConversion  OutDataTypeStr=fixdt_type_speed
  Data Type Conversion{3..4,44..45,52..53} (6 alike) : DataTypeConversion  OutDataTypeStr=fixdt_type_dq_currents
  Data Type Conversion30 : DataTypeConversion  OutDataTypeStr=fixdt_type_speed
  Data Type Conversion{32..36,38} (6 alike) : DataTypeConversion  OutDataTypeStr=fixdt_type_vsd
  Data Type Conversion37 : DataTypeConversion  OutDataTypeStr=boolean
  Data Type Conversion39 : DataTypeConversion  OutDataTypeStr=fixdt(1,18,14)
  Data Type Conversion40 : DataTypeConversion  OutDataTypeStr=fixdt_type_voltage
  Data Type Conversion{8..9,41..42,46..49} (8 alike) : DataTypeConversion  OutDataTypeStr=fixdt_type_dqxy_voltages
  Data Type Conversion54 : DataTypeConversion  OutDataTypeStr=fixdt_type_max_current
  Data Type Conversion{60..64} (5 alike) : DataTypeConversion  OutDataTypeStr=fixdt_type_lambda
  Data Type Conversion65 : DataTypeConversion  OutDataTypeStr=uint32
  Data Type Conversion67 : DataTypeConversion  OutDataTypeStr=fixdt(1,18,14)
  Delay : Delay  DelayLength=4
  Gain1 : Gain  Gain=0.5
  Mux2 : Mux
  Mux3 : Mux
  Mux6 : Mux  Inputs=12
  Mux7 : Mux  Inputs=5
  Mux8 : Mux  Inputs=2
  Mux9 : Mux  Inputs=2
  Pulse Generator1 : DiscretePulseGenerator  PulseType=Time based  Period=t_ADC  PulseWidth=5
  Rate Transition{1,5,8..9,60..61} (6 alike) : RateTransition  InitialCondition=1  OutPortSampleTime=t_clock
  Rate Transition{2..4,6..7,10..59,62..66} (60 alike) : RateTransition  OutPortSampleTime=t_clock
  Sawtooth Generator : SignalGenerator  WaveForm=sawtooth  Amplitude=2*pi  Frequency=2*pi*f  Units=rad/sec
  Scope : Scope  NumInputPorts=5
  Scope1 : Scope  NumInputPorts=5
  Scope2 : Scope  NumInputPorts=5
  Sum : Sum  Inputs=|+-
  Terminator{4,7..15} (10 alike) : Terminator
  uz_6_ph_mpc_delay_comp : Subsystem  TreatAsAtomicUnit=on
  uz_6ph_mpc_costs_and_optimization : Subsystem  TreatAsAtomicUnit=on
  uz_6ph_mpc_prediction : Subsystem  TreatAsAtomicUnit=on
  uz_6ph_mpc_pu_voltages_vsd : Subsystem  TreatAsAtomicUnit=on
  uz_park_transformation : Subsystem  TreatAsAtomicUnit=on
  uz_vsd_6ph_30deg : Subsystem  TreatAsAtomicUnit=on
  id_pred_pu_AXI : Outport
  iq_pred_pu_AXI : Outport  Port=2
  ix_pred_pu_AXI : Outport  Port=3
  iy_pred_pu_AXI : Outport  Port=4
  pu_ud_AXI : Outport  Port=5
  voltage_triggers : Outport  Port=6
  pu_uq_AXI : Outport  Port=7
  pu_ux_AXI : Outport  Port=8
  calc_done : Outport  Port=9
  Out10 : Outport  Port=10
  Out11 : Outport  Port=11
  Out1 : Outport  Port=12
  wires:
  Constant4/1 -> Data Type Conversion20/1
  Data Type Conversion47/1 -> Rate Transition47/1
  Rate Transition8/1 -> uz_6ph_mpc_pu_voltages_vsd/4(index)
  uz_6ph_mpc_prediction/5(id_pred_pu_AXI) -> id_pred_pu_AXI/1
  In2/1 -> Data Type Conversion33/1
  Mux8/1 -> Scope2/1
  uz_vsd_6ph_30deg/3(x1) -> [ix_pu]
  uz_6_ph_mpc_delay_comp/4(iy_delay_pu) -> [iy_delay_pu], Mux2/4
  [park_done_trigger] -> uz_6ph_mpc_prediction/20(adc_trigger)
  Data Type Conversion36/1 -> Rate Transition36/1
  [opt_index] -> Data Type Conversion59/1
  Rate Transition59/1 -> uz_6ph_mpc_costs_and_optimization/2(iq_ref_pu_AXI)
  Rate Transition25/1 -> uz_6ph_mpc_prediction/1(id_pu)
  Rate Transition6/1 -> uz_6_ph_mpc_delay_comp/5(vd_pu)
  Data Type Conversion7/1 -> Rate Transition8/1
  uz_vsd_6ph_30deg/8(alpha_AXI) -> Terminator8/1
  Data Type Conversion8/1 -> Rate Transition6/1
  uz_6ph_mpc_costs_and_optimization/7(G5) -> Mux6/6
  uz_6ph_mpc_prediction/8(iy_pred_pu_AXI) -> iy_pred_pu_AXI/1
  [opt_index] -> Data Type Conversion10/1
  uz_vsd_6ph_30deg/5(z1) -> Terminator4/1
  Rate Transition24/1 -> uz_6_ph_mpc_delay_comp/14(Ts_times_ZB_over_Ly_AXI)
  uz_6ph_mpc_costs_and_optimization/15(costs) -> Scope2/5
  Data Type Conversion28/1 -> Rate Transition28/1
  Rate Transition44/1 -> uz_6ph_mpc_prediction/3(ix_pu)
  uz_6ph_mpc_pu_voltages_vsd/4(pu_uy) -> Mux9/2, [uy_pu]
  uz_6ph_mpc_costs_and_optimization/11(G9) -> Mux6/10
  uz_6ph_mpc_pu_voltages_vsd/9(voltages_done) -> [voltages_done]  "calc_done"
  [ix_delay_pu] -> Data Type Conversion31/1
  [optimization_done] -> Mux7/5  "opt_done"
  Rate Transition57/1 -> uz_6ph_mpc_costs_and_optimization/1(id_ref_pu_AXI)
  [uy_pu] -> Data Type Conversion47/1
  uz_6ph_mpc_costs_and_optimization/4(G2) -> Mux6/3
  [uq_pu] -> Data Type Conversion49/1
  [ix_pu] -> Data Type Conversion/1
  Constant28/1 -> Data Type Conversion55/1
  Data Type Conversion2/1 -> Rate Transition2/1
  Constant12/1 -> Out11/1
  Rate Transition60/1 -> uz_6ph_mpc_costs_and_optimization/10(index)
  Constant2/1 -> Data Type Conversion13/1
  Rate Transition33/1 -> uz_vsd_6ph_30deg/3(c1)
  Data Type Conversion33/1 -> Rate Transition32/1
  Data Type Conversion31/1 -> Rate Transition44/1
  Data Type Conversion40/1 -> Rate Transition41/1
  Rate Transition10/1 -> uz_6ph_mpc_prediction/18(polepairs_AXI)
  [ux_pu] -> Data Type Conversion41/1
  Rate Transition52/1 -> uz_6ph_mpc_costs_and_optimization/7(ix_pred_pu)
  [id_pred_pu] -> Data Type Conversion52/1
  Rate Transition16/1 -> uz_6ph_mpc_prediction/16(Lq_over_LB_AXI)
  Rate Transition61/1 -> uz_6ph_mpc_costs_and_optimization/11(last_optim_index)
  uz_6ph_mpc_prediction/3(ix_pred_pu) -> Scope1/3, [ix_pred_pu]
  [ud_pu] -> Data Type Conversion8/1
  uz_6ph_mpc_prediction/2(iq_pred_pu) -> [iq_pred_pu], Scope1/2
  [trigger_prediction_done] -> uz_6ph_mpc_pu_voltages_vsd/8(trigger_prediction_done)
  uz_6ph_mpc_prediction/6(iq_pred_pu_AXI) -> iq_pred_pu_AXI/1
  Constant29/1 -> Data Type Conversion56/1
  Rate Transition37/1 -> uz_vsd_6ph_30deg/6(c2)
  uz_6ph_mpc_costs_and_optimization/6(G4) -> Mux6/5
  Data Type Conversion46/1 -> Rate Transition46/1
  Rate Transition4/1 -> uz_6_ph_mpc_delay_comp/2(iq_pu)
  Data Type Conversion34/1 -> Rate Transition33/1
  uz_6ph_mpc_pu_voltages_vsd/3(pu_ux) -> [ux_pu], Mux9/1
  Data Type Conversion54/1 -> Rate Transition54/1
  Data Type Conversion19/1 -> Rate Transition16/1
  Rate Transition46/1 -> uz_6ph_mpc_prediction/7(vx_pu)
  Constant16/1 -> Data Type Conversion30/1
  uz_6ph_mpc_prediction/4(iy_pred_pu) -> Scope1/4, [iy_pred_pu]
  [park_done_trigger] -> Mux7/1  "park_done"
  [voltages_done] -> uz_6_ph_mpc_delay_comp/19(trigger_voltages_done), Scope/4
  Rate Transition20/1 -> uz_6ph_mpc_prediction/9(omega_m_pu)
  Constant33/1 -> Data Type Conversion62/1
  Constant3/1 -> Data Type Conversion1/1
  [cos] -> uz_6ph_mpc_pu_voltages_vsd/3(cos_angle)
  Rate Transition53/1 -> uz_6ph_mpc_costs_and_optimization/6(iq_pred_pu)
  Rate Transition23/1 -> uz_6_ph_mpc_delay_comp/13(Ts_times_ZB_over_Lx_AXI)
  Data Type Conversion15/1 -> Rate Transition19/1
  [park_done_trigger] -> uz_6_ph_mpc_delay_comp/20(adc_trigger)
  In7/1 -> Rate Transition38/1
  Data Type Conversion9/1 -> Rate Transition7/1
  Rate Transition48/1 -> uz_6ph_mpc_prediction/5(vd_pu)
  Rate Transition9/1 -> uz_6ph_mpc_pu_voltages_vsd/10(last_opt_index)
  Rate Transition12/1 -> uz_6ph_mpc_prediction/13(Ts_times_ZB_over_Lx_AXI)
  uz_6ph_mpc_pu_voltages_vsd/6(pu_uq_AXI) -> pu_uq_AXI/1
  uz_6ph_mpc_prediction/1(id_pred_pu) -> [id_pred_pu], Scope1/1
  uz_6ph_mpc_costs_and_optimization/3(G1) -> Mux6/2
  [park_done_trigger] -> uz_6ph_mpc_pu_voltages_vsd/7(trigger_adc)
  [index] -> Data Type Conversion66/1, Data Type Conversion7/1
  uz_6_ph_mpc_delay_comp/5(id_delay_pu_AXI) -> Mux3/1
  Constant31/1 -> Data Type Conversion60/1
  [index] -> Data Type Conversion65/1
  [index_voltage] -> Mux8/2
  Data Type Conversion50/1 -> Rate Transition52/1
  Data Type Conversion38/1 -> Rate Transition37/1
  Data Type Conversion3/1 -> Rate Transition3/1
  Constant21/1 -> Data Type Conversion18/1
  uz_6_ph_mpc_delay_comp/6(iq_delay_pu_AXI) -> Mux3/2
  In4/1 -> Data Type Conversion35/1
  Data Type Conversion43/1 -> Rate Transition21/1
  uz_park_transformation/5(sin) -> [sin]
  uz_6ph_mpc_pu_voltages_vsd/5(pu_ud_AXI) -> pu_ud_AXI/1
  Constant22/1 -> Data Type Conversion19/1
  Pulse Generator1/1 -> Data Type Conversion37/1
  Rate Transition21/1 -> uz_6ph_mpc_prediction/4(iy_pu)
  Data Type Conversion58/1 -> Rate Transition59/1
  uz_6_ph_mpc_delay_comp/2(iq_delay_pu) -> [iq_delay_pu], Mux2/2
  uz_6ph_mpc_costs_and_optimization/9(G7) -> Mux6/8
  Data Type Conversion23/1 -> Rate Transition23/1
  Mux6/1 -> [opt_gates]
  uz_6ph_mpc_costs_and_optimization/14(opt_done) -> [optimization_done]  "optimization done"
  uz_6ph_mpc_costs_and_optimization/8(G6) -> Mux6/7
  [id_delay_pu] -> Data Type Conversion44/1
  Rate Transition35/1 -> uz_vsd_6ph_30deg/1(a1)
  Data Type Conversion45/1 -> Rate Transition45/1
  Data Type Conversion59/1 -> Rate Transition61/1
  Constant35/1 -> Data Type Conversion64/1
  Constant17/1 -> Data Type Conversion14/1
  uz_6_ph_mpc_delay_comp/1(id_delay_pu) -> [id_delay_pu], Mux2/1
  Data Type Conversion63/1 -> Rate Transition65/1
  Mux2/1 -> Scope/1
  Data Type Conversion/1 -> Rate Transition39/1
  Rate Transition38/1 -> Data Type Conversion67/1
  Data Type Conversion26/1 -> Rate Transition27/1
  Rate Transition17/1 -> uz_6ph_mpc_prediction/17(psi_pm_over_psiB_AXI)
  uz_park_transformation/6(cos) -> [cos]
  Constant32/1 -> Data Type Conversion61/1
  Rate Transition40/1 -> Data Type Conversion39/1
  Rate Transition58/1 -> uz_vsd_6ph_30deg/7(pu_conv_valid)
  Data Type Conversion62/1 -> Rate Transition64/1
  Data Type Conversion4/1 -> Rate Transition4/1
  Rate Transition18/1 -> uz_6ph_mpc_prediction/11(Ts_times_ZB_over_Ld_AXI)
  Mux9/1 -> Scope2/3
  Data Type Conversion12/1 -> Rate Transition11/1
  uz_6ph_mpc_prediction/10(index) -> Scope1/5, [index]
  Rate Transition55/1 -> uz_6ph_mpc_costs_and_optimization/3(ix_ref_pu_AXI)
  Data Type Conversion51/1 -> Rate Transition50/1
  Data Type Conversion52/1 -> Rate Transition51/1
  uz_6ph_mpc_prediction/9(prediction_done) -> [trigger_prediction_done]
  Rate Transition64/1 -> uz_6ph_mpc_costs_and_optimization/14(lambda_x_AXI)
  In5/1 -> Data Type Conversion36/1
  Rate Transition63/1 -> uz_6ph_mpc_costs_and_optimization/13(lambda_q_AXI)
  Rate Transition7/1 -> uz_6_ph_mpc_delay_comp/6(vq_pu)
  uz_6ph_mpc_costs_and_optimization/13(G11) -> Mux6/12
  Constant27/1 -> Data Type Conversion58/1
  Data Type Conversion37/1 -> Rate Transition58/1
  [ux_pu] -> Data Type Conversion46/1
  Rate Transition14/1 -> uz_6ph_mpc_prediction/14(Ts_times_ZB_over_Ly_AXI)
  Rate Transition22/1 -> uz_6_ph_mpc_delay_comp/10(Rs_over_ZB_AXI)
  Rate Transition51/1 -> uz_6ph_mpc_costs_and_optimization/5(id_pred_pu)
  Data Type Conversion53/1 -> Rate Transition53/1
  uz_6ph_mpc_costs_and_optimization/5(G3) -> Mux6/4
  uz_6ph_mpc_costs_and_optimization/10(G8) -> Mux6/9
  [index] -> Rate Transition60/1
  [iy_pred_pu] -> Data Type Conversion51/1
  Rate Transition62/1 -> uz_6ph_mpc_costs_and_optimization/12(lambda_d_AXI)
  Data Type Conversion55/1 -> Rate Transition55/1
  [uq_pu] -> Data Type Conversion9/1
  [sin] -> uz_6ph_mpc_pu_voltages_vsd/2(sin_angle)
  Data Type Conversion32/1 -> Rate Transition35/1
  Data Type Conversion29/1 -> Rate Transition31/1
  Constant39/1 -> Data Type Conversion57/1
  Delay/1 -> Scope2/2
  Mux7/1 -> Delay/1
  Rate Transition47/1 -> uz_6ph_mpc_prediction/8(vy_pu)
  Data Type Conversion13/1 -> Rate Transition13/1
  uz_vsd_6ph_30deg/4(y1) -> [iy_pu]
  Sawtooth Generator/1 -> Sum/2
  Constant14/1 -> Data Type Conversion27/1
  Data Type Conversion57/1 -> Rate Transition57/1
  [voltages_done] -> Mux7/2  "voltages_done"
  Constant34/1 -> Data Type Conversion63/1
  uz_vsd_6ph_30deg/7(vsd_done) -> uz_park_transformation/4(trigger)
  [trigger_prediction_done] -> Mux7/4  "prediction_done"
  Constant30/1 -> Data Type Conversion23/1
  Data Type Conversion60/1 -> Rate Transition62/1
  Data Type Conversion65/1 -> Mux8/1
  Constant36/1 -> Data Type Conversion24/1
  Data Type Conversion14/1 -> Rate Transition18/1
  [iq_pred_pu] -> Data Type Conversion53/1
  Rate Transition5/1 -> uz_6ph_mpc_pu_voltages_vsd/6(index_AXI)
  uz_6ph_mpc_costs_and_optimization/1(opt_index) -> [opt_index]  "result"
  Constant26/1 -> Data Type Conversion40/1
  Data Type Conversion24/1 -> Rate Transition24/1
  Rate Transition56/1 -> uz_6ph_mpc_costs_and_optimization/4(iy_ref_pu_AXI)
  uz_park_transformation/1(y1) -> [id_pu]
  [opt_index] -> Scope2/4
  Data Type Conversion67/1 -> uz_park_transformation/3(angle_el)
  Constant5/1 -> Data Type Conversion21/1
  Data Type Conversion1/1 -> Rate Transition1/1
  [iq_pu] -> Data Type Conversion4/1
  Rate Transition66/1 -> uz_6ph_mpc_costs_and_optimization/16(lambda_u_AXI)
  [ud_pu] -> Data Type Conversion48/1
  Rate Transition26/1 -> uz_6_ph_mpc_delay_comp/15(Ld_over_LB_AXI)
  uz_6ph_mpc_costs_and_optimization/12(G10) -> Mux6/11
  uz_6ph_mpc_prediction/7(ix_pred_pu_AXI) -> ix_pred_pu_AXI/1
  uz_6_ph_mpc_delay_comp/9(delay_comp_done) -> [delay_comp_done], Scope/3
  uz_park_transformation/2(y2) -> [iq_pu]
  uz_6ph_mpc_pu_voltages_vsd/10(index_voltage) -> [index_voltage]
  Rate Transition28/1 -> uz_6_ph_mpc_delay_comp/17(psi_pm_over_psiB_AXI)
  Rate Transition43/1 -> uz_6_ph_mpc_delay_comp/8(vy_pu)
  [index] -> Scope/5
  Constant15/1 -> Data Type Conversion12/1
  Data Type Conversion61/1 -> Rate Transition63/1
  Data Type Conversion10/1 -> Rate Transition9/1
  Rate Transition50/1 -> uz_6ph_mpc_costs_and_optimization/8(iy_pred_pu)
  [iy_pu] -> Data Type Conversion2/1
  Constant37/1 -> Data Type Conversion25/1
  Data Type Conversion48/1 -> Rate Transition48/1
  uz_6ph_mpc_pu_voltages_vsd/1(pu_ud) -> [ud_pu]
  Rate Transition54/1 -> uz_6ph_mpc_costs_and_optimization/9(max_current_pu_AXI)
  uz_vsd_6ph_30deg/12(z1_AXI) -> Terminator12/1
  Rate Transition3/1 -> uz_6_ph_mpc_delay_comp/1(id_pu)
  Data Type Conversion39/1 -> uz_park_transformation/5(factor_angle_el_AXI)
  Rate Transition11/1 -> uz_6ph_mpc_prediction/10(Rs_over_ZB_AXI)
  Rate Transition41/1 -> uz_6ph_mpc_pu_voltages_vsd/1(v_DC_pu)
  uz_6ph_mpc_pu_voltages_vsd/2(pu_uq) -> [uq_pu]
  [delay_comp_done] -> Mux7/3  "delay_comp_done"
  Rate Transition42/1 -> uz_6_ph_mpc_delay_comp/7(vx_pu)
  Rate Transition45/1 -> uz_6ph_mpc_prediction/2(iq_pu)
  uz_vsd_6ph_30deg/11(y_AXI) -> Terminator11/1
  Rate Transition49/1 -> uz_6ph_mpc_prediction/6(vq_pu)
  Data Type Conversion49/1 -> Rate Transition49/1
  [voltages_done] -> uz_6ph_mpc_prediction/19(trigger_voltages_done)
  Constant19/1 -> Data Type Conversion16/1
  Data Type Conversion27/1 -> Rate Transition17/1
  Data Type Conversion44/1 -> Rate Transition25/1
  Data Type Conversion30/1 -> Rate Transition20/1
  Data Type Conversion17/1 -> Rate Transition14/1
  Constant13/1 -> Data Type Conversion11/1
  Rate Transition15/1 -> uz_6ph_mpc_prediction/15(Ld_over_LB_AXI)
  Rate Transition30/1 -> uz_6_ph_mpc_delay_comp/12(Ts_times_ZB_over_Lq_AXI)
  uz_6_ph_mpc_delay_comp/3(ix_delay_pu) -> [ix_delay_pu], Mux2/3
  Rate Transition1/1 -> uz_6ph_mpc_pu_voltages_vsd/5(index_select)
  uz_park_transformation/7(park_done) -> [park_done_trigger]  "calc_done"
  Constant11/1 -> Data Type Conversion54/1
  Data Type Conversion16/1 -> Rate Transition12/1
  Data Type Conversion66/1 -> Rate Transition5/1
  Data Type Conversion64/1 -> Rate Transition66/1
  Constant18/1 -> Data Type Conversion15/1
  Sum/1 -> Gain1/1
  Rate Transition13/1 -> uz_6_ph_mpc_delay_comp/18(polepairs_AXI)
  uz_6_ph_mpc_delay_comp/8(iy_delay_pu_AXI) -> Mux3/4
  Rate Transition34/1 -> uz_vsd_6ph_30deg/4(a2)
  Constant10/1 -> Data Type Conversion28/1
  uz_park_transformation/3(y1_AXI) -> Terminator14/1
  Constant25/1 -> Rate Transition40/1
  Data Type Conversion18/1 -> Rate Transition15/1
  uz_vsd_6ph_30deg/1(alpha) -> uz_park_transformation/1(u1)
  [ix_pred_pu] -> Data Type Conversion50/1
  uz_6ph_mpc_costs_and_optimization/2(G0) -> Mux6/1
  Data Type Conversion41/1 -> Rate Transition42/1
  Data Type Conversion35/1 -> Rate Transition34/1
  [iq_delay_pu] -> Data Type Conversion45/1
  uz_vsd_6ph_30deg/10(x_AXI) -> Terminator10/1
  uz_6_ph_mpc_delay_comp/7(ix_delay_pu_AXI) -> Mux3/3
  [delay_comp_done] -> uz_6ph_mpc_pu_voltages_vsd/9(trigger_delay_comp_done)
  Data Type Conversion56/1 -> Rate Transition56/1
  [id_pu] -> Data Type Conversion3/1
  Constant20/1 -> Data Type Conversion17/1
  In3/1 -> Data Type Conversion34/1
  Rate Transition32/1 -> uz_vsd_6ph_30deg/2(b1)
  [iy_delay_pu] -> Data Type Conversion43/1
  Data Type Conversion11/1 -> Rate Transition10/1
  uz_vsd_6ph_30deg/13(z2_AXI) -> Terminator13/1
  uz_vsd_6ph_30deg/2(beta) -> uz_park_transformation/2(u2)
  Data Type Conversion25/1 -> Rate Transition26/1
  Constant24/1 -> Sum/1
  Data Type Conversion20/1 -> Rate Transition22/1
  Rate Transition31/1 -> uz_6_ph_mpc_delay_comp/9(omega_m_pu)
  uz_park_transformation/4(y2_AXI) -> Terminator15/1
  Mux3/1 -> Scope/2
  Data Type Conversion42/1 -> Rate Transition43/1
  Data Type Conversion22/1 -> Rate Transition30/1
  Constant7/1 -> Data Type Conversion22/1
  Rate Transition39/1 -> uz_6_ph_mpc_delay_comp/3(ix_pu)
  Constant23/1 -> Data Type Conversion29/1
  Rate Transition29/1 -> uz_6_ph_mpc_delay_comp/11(Ts_times_ZB_over_Ld_AXI)
  uz_vsd_6ph_30deg/9(beta_AXI) -> Terminator9/1
  Rate Transition2/1 -> uz_6_ph_mpc_delay_comp/4(iy_pu)
  Data Type Conversion21/1 -> Rate Transition29/1
  [uy_pu] -> Data Type Conversion42/1
  Rate Transition36/1 -> uz_vsd_6ph_30deg/5(b2)
  Rate Transition27/1 -> uz_6_ph_mpc_delay_comp/16(Lq_over_LB_AXI)
  Rate Transition65/1 -> uz_6ph_mpc_costs_and_optimization/15(lambda_y_AXI)
  uz_vsd_6ph_30deg/6(z2) -> Terminator7/1
  Constant38/1 -> Data Type Conversion26/1
  Rate Transition19/1 -> uz_6ph_mpc_prediction/12(Ts_times_ZB_over_Lq_AXI)
  [trigger_prediction_done] -> uz_6ph_mpc_costs_and_optimization/17(trigger)
  uz_6ph_mpc_pu_voltages_vsd/11(voltage_triggers) -> voltage_triggers/1
  In6/1 -> Data Type Conversion38/1
  In1/1 -> Data Type Conversion32/1
  uz_6ph_mpc_pu_voltages_vsd/7(pu_ux_AXI) -> pu_ux_AXI/1
  Constant42/1 -> Out10/1
  uz_6ph_mpc_pu_voltages_vsd/8(pu_uy_AXI) -> calc_done/1  "calc_done"
  [opt_gates] -> Out1/1
